simulink model "Pur_Pursuit"  (R2022a)
settings: Solver=FixedStepAuto  StartTime=0.0  StopTime=T  FixedStep=Te  RelTol=1e-3
undefined symbols (not defined in the file): d, DiscIntNeverNeededParam, L, psi, Te, v, xg, yg
settings Model: Creator=leonj  LastModifiedBy=leonj

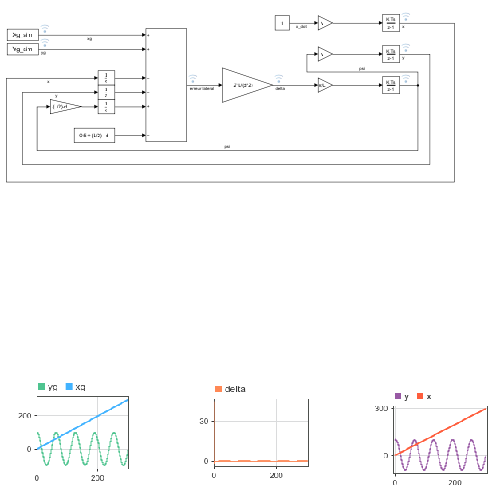
[thumbnail: Simulink's stored preview of the top-level diagram]
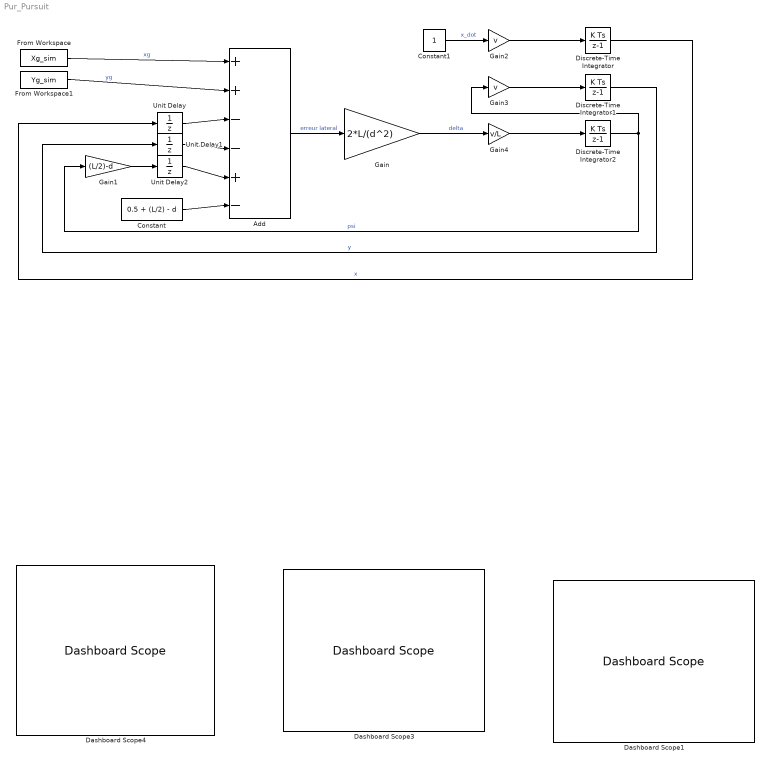
== system Pur_Pursuit ==
  Add : Sum  Inputs=++|--+|-
  Constant : Constant  Value=0.5 + (L/2) - d  SampleTime=Te
  Constant1 : Constant  SampleTime=Te
  Dashboard Scope1 : DashboardScope
  Dashboard Scope3 : DashboardScope
  Dashboard Scope4 : DashboardScope  Ymin=-10  Ymax=10
  Discrete-Time Integrator : DiscreteIntegrator  gainval=1/v  InitialCondition=xg  SampleTime=Te  ICPrevOutput=DiscIntNeverNeededParam  ICPrevScaledInput=DiscIntNeverNeededParam
  Discrete-Time Integrator1 : DiscreteIntegrator  gainval=1/v  InitialCondition=yg  SampleTime=Te  ICPrevOutput=DiscIntNeverNeededParam  ICPrevScaledInput=DiscIntNeverNeededParam
  Discrete-Time Integrator2 : DiscreteIntegrator  InitialCondition=psi  SampleTime=Te  ICPrevOutput=DiscIntNeverNeededParam  ICPrevScaledInput=DiscIntNeverNeededParam
  From Workspace : FromWorkspace  VariableName=Xg_sim  SampleTime=Te
  From Workspace1 : FromWorkspace  VariableName=Yg_sim  SampleTime=Te
  Gain : Gain  Gain=2*L/(d^2)
  Gain1 : Gain  Gain=(L/2)-d
  Gain2 : Gain  Gain=v
  Gain3 : Gain  Gain=v
  Gain4 : Gain  Gain=v/L
  Unit Delay : UnitDelay  SampleTime=Te  HasFrameUpgradeWarning=on
  Unit Delay1 : UnitDelay  SampleTime=Te  HasFrameUpgradeWarning=on
  Unit Delay2 : UnitDelay  SampleTime=Te  HasFrameUpgradeWarning=on
  wires:
  From Workspace/1 -> Add/1  "xg"
  From Workspace1/1 -> Add/2  "yg"
  Discrete-Time Integrator2/1 -> Gain1/1, Gain3/1  "psi"
  Add/1 -> Gain/1  "erreur lateral"
  Unit Delay/1 -> Add/3
  Unit Delay1/1 -> Add/4
  Unit Delay2/1 -> Add/5
  Gain1/1 -> Unit Delay2/1
  Constant/1 -> Add/6
  Gain2/1 -> Discrete-Time Integrator/1
  Gain3/1 -> Discrete-Time Integrator1/1
  Gain4/1 -> Discrete-Time Integrator2/1
  Gain/1 -> Gain4/1  "delta"
  Constant1/1 -> Gain2/1  "x_dot"
  Discrete-Time Integrator1/1 -> Unit Delay1/1  "y"
  Discrete-Time Integrator/1 -> Unit Delay/1  "x"
